simulink model "dc_mot2"  (R2019b)
settings: Solver=VariableStepAuto  StartTime=0.0  StopTime=1  RelTol=1e-3
InitFcn:
  | Ra = 1.2; % Armature resistance
  | La = 2.5e-3; %armature inductance
  | Kc = 0.35; %flux constant
  | J = 1e-3; % moment of inertia
  | %% Gains of the 2DOF PI current controller
  | alphac = 2*pi*500; %closed loop bandwidth
  | Kpc = alphac*La; % proportional gain
  | Kic = alphac*2*La; %integral gain
  | r = Kpc- Ra; %active resistance
  | Umax = 72; %saturation: upper limit
  | Umin = -72; %saturation lower limit
values from neighbouring files (symbols this model uses):
  b = [2 2]    [test.m]
settings Model: Creator=srikesh  LastModifiedBy=srikesh

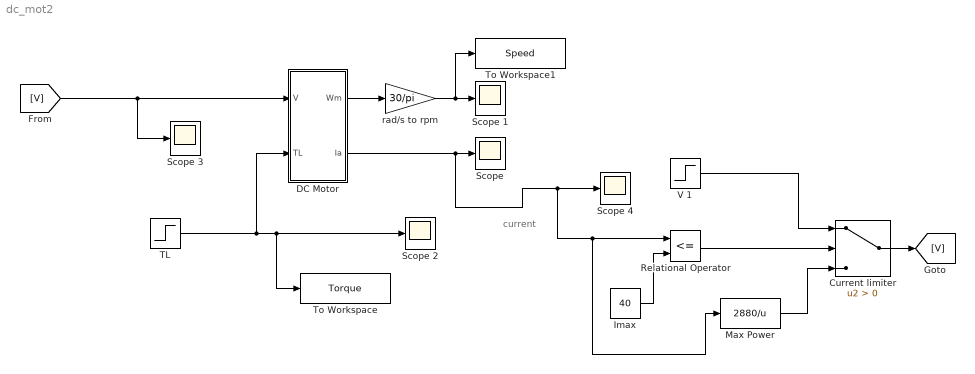
== system dc_mot2 ==
  note: current
  "Current limiter " : Switch  Criteria=u2 > Threshold
  "DC Motor " : Subsystem  mask{Ra=.1472, Ke=1.27, Kt=.9852}
      mask prompts: Ra "Ra(Ohm)"; Ke "Ke(V-s)"; Kt "Kt(N-m/A)"
  Imax : Constant  Value=40
  Max Power : Fcn  Expr=2880/u
  Relational Operator : RelationalOperator  Operator=<=  OutDataTypeStr=boolean  RndMeth=Simplest
  Scope {,1..4} (5 alike) : Scope
  TL : Step  Time=.1  Before=2  After=42  SampleTime=0
  To Workspace : ToWorkspace  VariableName=Torque  SaveFormat=Timeseries  SampleTime=-1
  To Workspace1 : ToWorkspace  VariableName=Speed  SaveFormat=Timeseries  SampleTime=-1
  V 1 : Step  Time=.1  Before=72  After=72  SampleTime=0
  "rad/s to rpm " : Gain  Gain=30/pi
  wires:
  "rad/s to rpm "/1 -> To Workspace1/1, Scope 1/1
  TL/1 -> Scope 2/1, To Workspace/1, "DC Motor "/2("TL ")
  "DC Motor "/1("Wm ") -> "rad/s to rpm "/1
  [V] -> Scope 3/1, "DC Motor "/1("V ")
  "DC Motor "/2(Ia) -> Relational Operator/1, Max Power/1, Scope 4/1, "Scope "/1
  Relational Operator/1 -> "Current limiter "/2
  V 1/1 -> "Current limiter "/1
  "Current limiter "/1 -> [V]
  Max Power/1 -> "Current limiter "/3
  Imax/1 -> Relational Operator/2

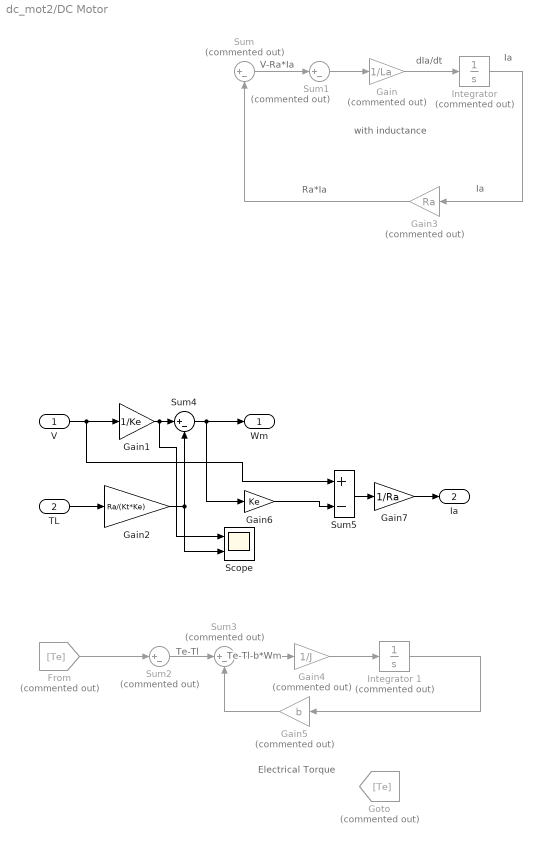
== system dc_mot2/DC Motor  ==
  note: with inductance
  note: Electrical Torque
  note: Te-Tl-b*Wm
  note: Te-Tl
  note: Ia
  note: Ra*Ia
  note: V-Ra*Ia
  note: dIa/dt
  note: Ia
  "V " : Inport
  "TL " : Inport  Port=2
  From : From  Commented=on  GotoTag=Te
  Gain : Gain  Commented=on  Gain=1/La
  Gain1 : Gain  Gain=1/Ke
  Gain2 : Gain  Gain=Ra/(Kt*Ke)
  Gain3 : Gain  Commented=on  Gain=Ra
  Gain4 : Gain  Commented=on  Gain=1/J
  Gain5 : Gain  Commented=on  Gain=b
  Gain6 : Gain  Gain=Ke
  Gain7 : Gain  Gain=1/Ra
  "Goto " : Goto  Commented=on  GotoTag=Te
  "Integrator " : Integrator  Commented=on
  Integrator 1 : Integrator  Commented=on
  Scope : Scope  NumInputPorts=2
  Sum{,1..3} (4 alike) : Sum  Commented=on  Inputs=|+-
  Sum4 : Sum  Inputs=|+-
  Sum5 : Sum  Inputs=+-
  "Wm " : Outport
  Ia : Outport  Port=2
  wires:
  Sum3/1 -> Gain4/1
  Sum2/1 -> Sum3/1
  From/1 -> Sum2/1
  Gain4/1 -> Integrator 1/1
  Gain5/1 -> Sum3/2
  Gain3/1 -> Sum/2
  Integrator 1/1 -> Gain5/1
  Sum1/1 -> Gain/1
  Sum/1 -> Sum1/1
  "Integrator "/1 -> Gain3/1
  Gain/1 -> "Integrator "/1
  "V "/1 -> Sum5/1, Gain1/1
  Gain1/1 -> Scope/1, Sum4/1
  "TL "/1 -> Gain2/1
  Gain2/1 -> Sum4/2, Scope/2
  Sum4/1 -> Gain6/1, "Wm "/1
  Gain6/1 -> Sum5/2
  Gain7/1 -> Ia/1
  Sum5/1 -> Gain7/1
